simulink model "simulink_1avrilhaha"  (R2024a)
settings: Solver=VariableStepAuto  StartTime=0.0  StopTime=700  RelTol=1e-3
libraries: simulink_extras x1
settings Model: Creator=sabri  LastModifiedBy=sabri

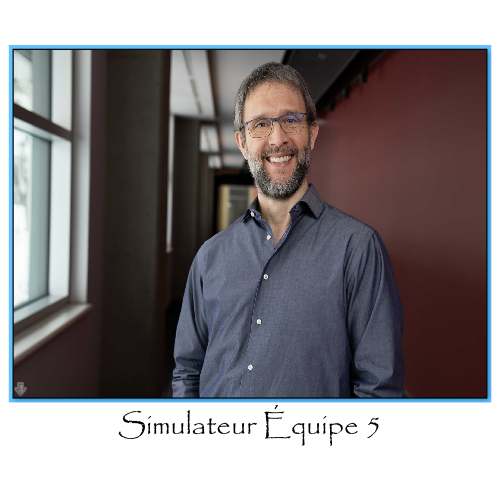
[thumbnail: Simulink's stored preview of the top-level diagram]
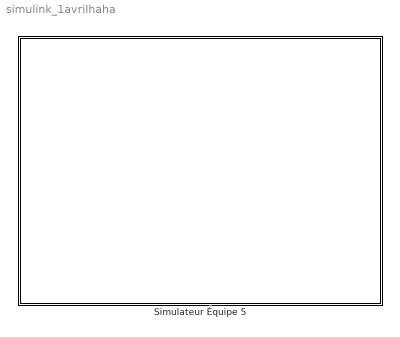
== system simulink_1avrilhaha ==
  Simulateur Équipe 5 : Subsystem  mask{V_2=5, V_1=1.8, R_1=3300, R_g=5600, R_f=6300, T_0=298.15, RT_0=10000, B=3782, Enregistrement=on, Consigne=30}
      mask prompts: V_2 "Tension d'alimentation (V)"; V_1 "Tension d'alimentation de la branche positive de l'ampli-op (V)"; R_1 "Résistance de la branche négative de l'ampli-op (Ω)"; R_g "Résistance en parallèle avec la thermitance (Ω)"; R_f "Résistance du trimpot (Ω)"; T_0 "Température de référence de la thermistance (K)"; RT_0 "Résistance de référence de la thermistance (Ω)"; B "Valeur beta de la thermistance"; Enregistrement "Enregistrement des données"; Consigne "Température désirée"
      mask DialogControl Container3 Prompt: Guide d'utilisateur
      mask DialogControl Control2 Prompt: Voici le simulateur thermique de l'équipe 5. Vous pouvez modifier les valeurs des différents paramètres du prototype si-dessus et choisir la température désirée.
      mask DialogControl Container4 Prompt: Paramètres du prototype
      mask Display: image('4e9b43_37b74c7254004fa5961c1584dfcae1f1~mv2.jpg');

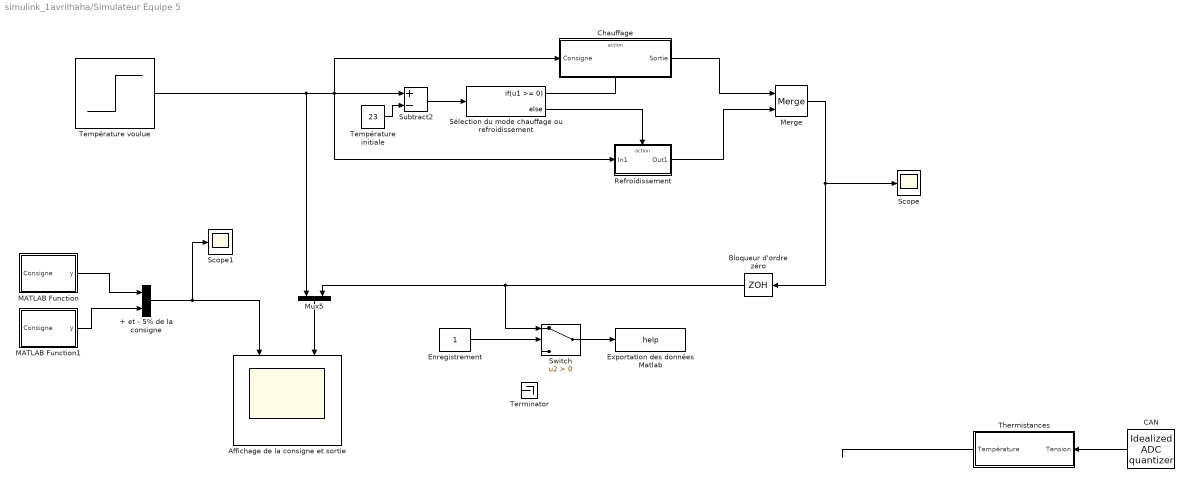
== system simulink_1avrilhaha/Simulateur Équipe 5 ==
  + et - 5% de la consigne : Mux  Inputs=2
  Affichage de la consigne et sortie : Scope  NumInputPorts=2
  Bloqueur d'ordre zéro : ZeroOrderHold  SampleTime=0.5
  CAN : simulink_extras/Additional Discrete/Idealized ADC quantizer  NumberOfConverterBits=10  Vmin=0  Vmax=50  OutputDataType=double  OutputNegativeValues=off
  Chauffage : Subsystem  TreatAsAtomicUnit=on
  Enregistrement : Constant
  Exportation des données Matlab : ToWorkspace  VariableName=help  SampleTime=0.5
  MATLAB Function : MATLAB Function  TreatAsAtomicUnit=on
  MATLAB Function1 : MATLAB Function  TreatAsAtomicUnit=on
  Merge : Merge
  Mux5 : Mux  Inputs=2
  Refroidissement : Subsystem  TreatAsAtomicUnit=on
  Scope : Scope
  Scope1 : Scope
  Subtract2 : Sum  Inputs=+-
  Switch : Switch  Criteria=u2 > Threshold  SaturateOnIntegerOverflow=off  InputSameDT=off
  Sélection du mode chauffage ou refroidissement : If  IfExpression=u1 >= 0
  Température initiale : Constant  Value=23
  Température voulue : Step  Time=0  Before=Consigne  After=Consigne  SampleTime=0
  Terminator : Terminator
  Thermistances : Subsystem
  wires:
  MATLAB Function1/1(y) -> + et - 5% de la consigne/2
  Subtract2/1 -> Sélection du mode chauffage ou refroidissement/1
  + et - 5% de la consigne/1 -> Scope1/1, Affichage de la consigne et sortie/1
  Température voulue/1 -> Refroidissement/1(In1), Chauffage/1(Consigne), Subtract2/1, Mux5/1
  Merge/1 -> Scope/1, Bloqueur d'ordre zéro/1
  MATLAB Function/1(y) -> + et - 5% de la consigne/1
  Refroidissement/1(Out1) -> Merge/2
  Sélection du mode chauffage ou refroidissement/2 -> Refroidissement/Action
  Mux5/1 -> Affichage de la consigne et sortie/2
  Sélection du mode chauffage ou refroidissement/1 -> Chauffage/Action
  Température initiale/1 -> Subtract2/2
  Bloqueur d'ordre zéro/1 -> Mux5/2, Switch/1
  ? -> CAN/1
  Thermistances/1(Température) -> ?
  CAN/1 -> Thermistances/1(Tension)
  Chauffage/1(Sortie) -> Merge/1
  Enregistrement/1 -> Switch/2
  Switch/1 -> Exportation des données Matlab/1

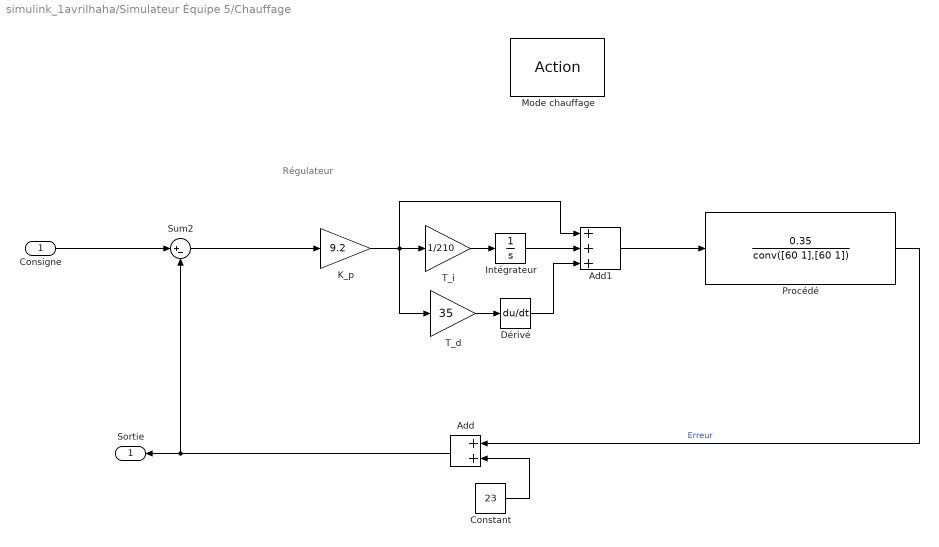
== system simulink_1avrilhaha/Simulateur Équipe 5/Chauffage ==
  note: Régulateur
  Consigne : Inport
  Mode chauffage : ActionPort  ActionPortLabel=if(u1 >= 0)
  Add : Sum
  Add1 : Sum  Inputs=+++
  Constant : Constant  Value=23
  Dérivé : Derivative
  Intégrateur : Integrator
  K_p : Gain  Gain=9.2
  Procédé : TransferFcn  Numerator=[0.35]  Denominator=conv([60 1],[60 1])
  Sum2 : Sum  Inputs=|+-
  T_d : Gain  Gain=35
  T_i : Gain  Gain=1/210
  Sortie : Outport
  wires:
  Sum2/1 -> K_p/1
  Intégrateur/1 -> Add1/2
  Add1/1 -> Procédé/1
  T_i/1 -> Intégrateur/1
  T_d/1 -> Dérivé/1
  Dérivé/1 -> Add1/3
  K_p/1 -> Add1/1, T_d/1, T_i/1
  Consigne/1 -> Sum2/1
  Add/1 -> Sortie/1, Sum2/2
  Procédé/1 -> Add/1  "Erreur"
  Constant/1 -> Add/2

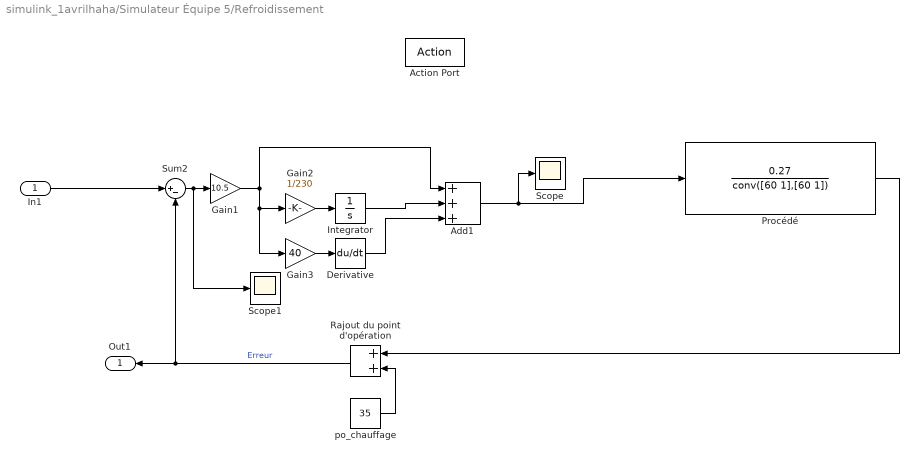
== system simulink_1avrilhaha/Simulateur Équipe 5/Refroidissement ==
  In1 : Inport
  Action Port : ActionPort  ActionPortLabel=else
  Add1 : Sum  Inputs=+++
  Derivative : Derivative
  Gain1 : Gain  Gain=10.5
  Gain2 : Gain  Gain=1/230
  Gain3 : Gain  Gain=40
  Integrator : Integrator
  Procédé : TransferFcn  Numerator=[0.27]  Denominator=conv([60 1],[60 1])
  Rajout du point d'opération : Sum
  Scope : Scope
  Scope1 : Scope
  Sum2 : Sum  Inputs=|+-
  po_chauffage : Constant  Value=35
  Out1 : Outport
  wires:
  Gain2/1 -> Integrator/1
  Gain3/1 -> Derivative/1
  Integrator/1 -> Add1/2
  Derivative/1 -> Add1/3
  Gain1/1 -> Add1/1, Gain3/1, Gain2/1
  Add1/1 -> Scope/1, Procédé/1
  Sum2/1 -> Scope1/1, Gain1/1
  In1/1 -> Sum2/1
  po_chauffage/1 -> Rajout du point d'opération/2
  Procédé/1 -> Rajout du point d'opération/1
  Rajout du point d'opération/1 -> Sum2/2, Out1/1  "Erreur"

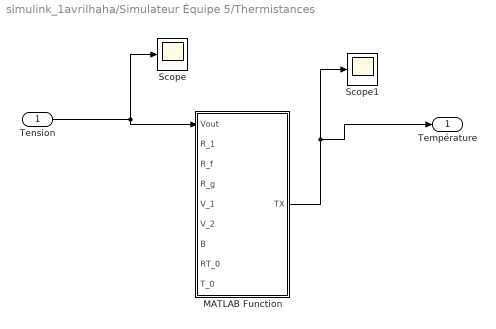
== system simulink_1avrilhaha/Simulateur Équipe 5/Thermistances ==
  Tension : Inport
  MATLAB Function : MATLAB Function  TreatAsAtomicUnit=on
  Scope : Scope
  Scope1 : Scope
  Température : Outport
  wires:
  Tension/1 -> Scope/1, MATLAB Function/1(Vout)
  MATLAB Function/1(TX) -> Scope1/1, Température/1

== matlab function simulink_1avrilhaha/Simulateur Équipe 5/MATLAB Function1 ==
  data: Consigne input; y output
function y = fcn(Consigne)

y = -0.05*Consigne;

== matlab function simulink_1avrilhaha/Simulateur Équipe 5/MATLAB Function ==
  data: Consigne input; y output
function y = fcn(Consigne)

y = 0.05*Consigne;

== matlab function simulink_1avrilhaha/Simulateur Équipe 5/Thermistances/MATLAB Function ==
  data: Vout input; TX output; R_1 input; R_f input; R_g input; V_1 input; V_2 input; B input; RT_0 input; T_0 input
function TX = fcn(Vout, R_1, R_f, R_g, V_1, V_2, B, RT_0, T_0)
    RT = ((R_f + R_1) * R_g * V_2) / (R_1 * (5*Vout/1023) + R_f * V_1) - R_g;
    TX = 1 / ((log(RT / RT_0) / B) + (1 / T_0)) - 273.15;
end
